simulink model "Base_Case_v1"  (R2021a)
settings: Solver=FixedStepDiscrete  StartTime=0.0  StopTime=24  FixedStep=Ts_Power  RelTol=1e-3
InitFcn:
  | %Simulation parameters
  | Ts_Power = 50e-6;
  | Ts_Control = 50e-6;
  | Ts_sec = 0.05;
  | 
  | %MV Grid parameters
  | U1n = 20e3;
  | f = 50;
  | omega = 2*pi*50;
  | 
  | 
  | %LCL filter parameters
  | L_t = 100e-6;
  | C = 173e-6;
  | L_s = 100e-6;
  | R_d = 0.086;
  | R_t = omega*L_t/100;
  | R_s = omega*L_s/100;
  | 
  | %Capacitance of the DC bus
  | Cdc = 5.88e-3;
  | Rdc = 0.00001;
  | 
  | %Coupling transformers parameters
  | U2n = 400;
  | Sn1 = 3e6;
  | 
  | %Primary Subestation parameters
  | Un = 110e3;
  | Sn = 30e6;
  | 
  | %Feeder parameters
  | Le_line_1 = 12; %length km
  | R_line_1 = (0.337)*Le_line_1; %Resistance ohms
  | X_line_1 = (0.358)*Le_line_1; %Reactance ohms
  | L_line_1 = X_line_1/omega;%Inductance H
  | 
  | Le_line_2 = 10; %length km
  | R_line_2 = (0.337)*Le_line_2; %Resistance ohms
  | X_line_2 = (0.358)*Le_line_2; %Reactance ohms
  | L_line_2 = X_line_2/omega; %Inductance H
  | 
  | %PLL parameters
  | K_p_pll = 1.8;
  | K_i_pll = 1.8/0.00251;
  | 
  | %Current control loop gains
  | tau_c = 3e-3;
  | L = L_t + L_s;
  | R =R_t + R_s;
  | Kp = L/tau_c;
  | Ki = R/tau_c;
  | 
  | %DC bus voltage control loop gains
  | tau_dc = 3*tau_c;
  | 
  | %Q-V primary control loop
  | RQ = 0.15; %Q-V regulation constant
  | 
  | %24-hours household profile pu
  | t_profile = [0:1:24].';
  | p_profile_h = [0.26 0.2 0.19 0.19 0.19 0.25 0.4 0.6 0.64 0.64 0.67 0.6 0.73 0.63 0.57 0.5 0.47 0.65 0.8 0.93 0.82 0.67 0.55 0.38 0.26].';
  | fdp_h = 0.87;
  | fi_h = acos(fdp_h);
  | q_profile_h = p_profile_h*tan(fi_h);
  | S_h = 3e6;
  | 
  | %24-hours industrial profile pu
  | p_profile_i = [0.33 0.32 0.29 0.32 0.37 0.45 0.67 0.88 1 0.99 1 0.79 0.83 0.83 0.83 0.8 0.55 0.65 0.5 0.46 0.41 0.4 0.36 0.36 0.33].';
  | fdp_i = 0.98;
  | fi_i = acos(fdp_h);
  | q_profile_i = p_profile_i*tan(fi_i);
  | S_i = 3e6;
  | 
  | %24-hours PV profile pu
  | p_profile_pv = [0 0 0 0 0 0 0 0 0 0.03 0.12 0.14 0.15 0.12 0.11 0.10 0.09 0.07 0.04 0 0 0 0 0 0].'*1/0.15;
  | S_pv = 6e6;
  | 
  | %24-hours WT profile pu
  | p_profile_wt = [0.9 0.9 1.1 1 0.9 1.1 1.25 1 0.9 0.8 0.9 0.9 1 0.8 1.5 1.3 1.2 1.2 1 0.7 1.2 0.9 1.3 1.4 0.9].'*1/1.5;
  | S_wt= 8e6;
undefined symbols (not defined in the file): DiscIntNeverNeededParam
libraries: spsThreePhaseSeriesRLCBranchLib x10, spsThreePhaseVIMeasurementLib x9, spsRMSLib x8, simulink x6, spsThreePhaseDynamicLoadLib x4, spsThreePhaseBreakerLib x2, spsThreePhaseTransformerTwoWindingsLib x2, spsThreePhaseSourceLib x1, spsPower3phInstantaneousLib x1, spspowerguiLib x1
settings Model: Creator=Manuel  LastModifiedBy=Manuel_Barragan

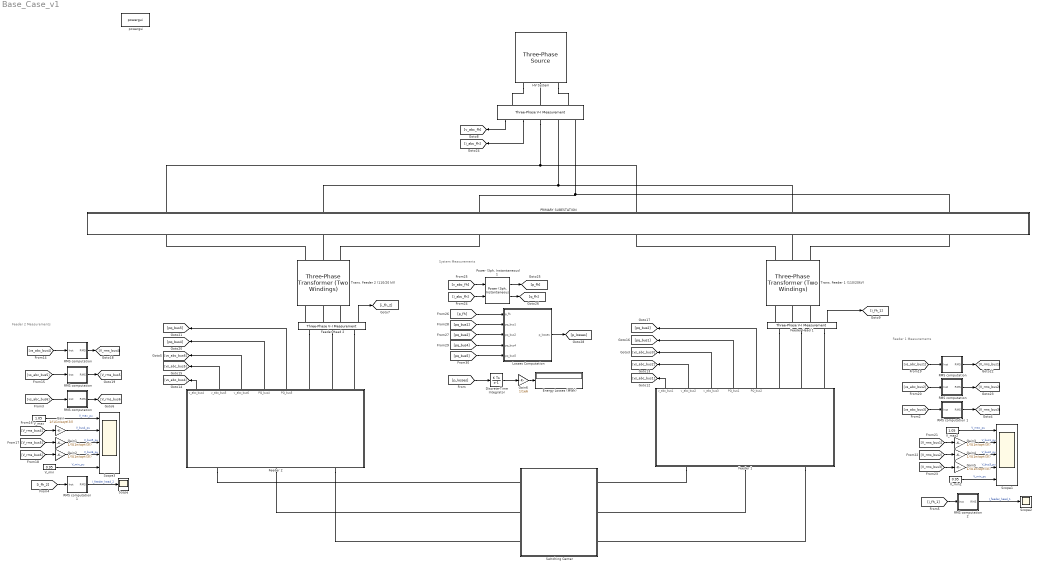
== system Base_Case_v1 ==
  note: Feeder 2 Measurements
  note: Feeder 1 Measurements
  note: System Measurements
  " " : spsThreePhaseVIMeasurementLib/Three-Phase V-I Measurement  VoltageMeasurement=phase-to-ground  SetLabelV=off  LabelV=Vabc  Vpu=off  VpuLL=off  CurrentMeasurement=yes  SetLabelI=off  LabelI=Iabc  Ipu=off  Pbase=100e6  Vbase=500e3  OutputType=Complex  PhasorSimulation=off  PSBequivalent=0
  Discrete-Time Integrator : DiscreteIntegrator  SampleTime=Ts_Control  ICPrevOutput=DiscIntNeverNeededParam  ICPrevScaledInput=DiscIntNeverNeededParam
  Energy Losses (MWh) : Display
  Feeder 1 : Subsystem
  Feeder 2 : Subsystem
  Feeder Head 1 : spsThreePhaseVIMeasurementLib/Three-Phase V-I Measurement  VoltageMeasurement=no  SetLabelV=off  LabelV=Vabc  Vpu=off  VpuLL=off  CurrentMeasurement=yes  SetLabelI=off  LabelI=Iabc  Ipu=off  Pbase=100e6  Vbase=500e3  OutputType=Complex  PhasorSimulation=off  PSBequivalent=0
  Feeder Head 2 : spsThreePhaseVIMeasurementLib/Three-Phase V-I Measurement  VoltageMeasurement=no  SetLabelV=off  LabelV=Vabc  Vpu=off  VpuLL=off  CurrentMeasurement=yes  SetLabelI=off  LabelI=Iabc  Ipu=off  Pbase=100e6  Vbase=500e3  OutputType=Complex  PhasorSimulation=off  PSBequivalent=0
  Gain{,1..5} (6 alike) : Gain  Gain=1/(U1n/sqrt(3))
  Gain6 : Gain  Gain=1/1e6
  HV System : spsThreePhaseSourceLib/Three-Phase Source  InternalConnection=Yg  VoltagePhases=off  Voltage=Un  PhaseAngle=0  Voltage_phases=[25e3 25e3 25e3]/sqrt(3)  PhaseAngles_phases=[0 -120 +120]  Frequency=f  NonIdealSource=off  SpecifyImpedance=on  Resistance=0.8929  Inductance=16.58e-3  ShortCircuitLevel=100e6  BaseVoltage=V  XRratio=7  BusType=swing  Pref=10e3  Qref=0  Prefabc=[10e3, 10e3, 10e3]  Qrefabc=[0, 0, 0]  Qmin=-inf  Qmax=inf
  Losses Computation : MATLAB Function  TreatAsAtomicUnit=on
  PRIMARY SUBESTATION : Subsystem
  "Power (3ph, Instantaneous)1" : spsPower3phInstantaneousLib/Power (3ph, Instantaneous)
  RMS computation : Subsystem
  "RMS computation " : Subsystem
  "RMS computation  " : Subsystem
  "RMS computation   " : Subsystem
  "RMS computation    " : Subsystem
  RMS computation  1 : Subsystem
  RMS computation  2 : Subsystem
  RMS computation 1 : Subsystem
  Scope : Scope
  Scope1 : Scope  NumInputPorts=5
  Scope2 : Scope
  Scope3 : Scope  NumInputPorts=5
  Switching Center : Subsystem
  Trans. Feeder 1 (110/20kV) : spsThreePhaseTransformerTwoWindingsLib/Three-Phase Transformer (Two Windings)  Winding1Connection=Yg  Winding2Connection=Yg  CoreType=Three single-phase transformers  SetSaturation=off  Hysteresis=off  DataFile='hysteresis'  SetInitialFlux=off  Measurements=None  UNITS=pu  NominalPower=[ Sn , f ]  Winding1=[ Un , 0.002 , 0.08 ]  Winding2=[ U1n , 0.002 , 0.08 ]  Rm=500  Lm=500  L0=0.5  Saturation=[ 0,0 ; 0.0024,1.2 ; 1.0,1.52 ]  InitialFluxes=[ 0.8 , -0.8 , 0.7 ]  BreakLoop=off  DiscreteSolver=Trapezoidal iterative  DataType=off  TransfoNumber=1
  Trans. Feeder 2 (110/20 kV) : spsThreePhaseTransformerTwoWindingsLib/Three-Phase Transformer (Two Windings)  Winding1Connection=Yg  Winding2Connection=Yg  CoreType=Three single-phase transformers  SetSaturation=off  Hysteresis=off  DataFile='hysteresis'  SetInitialFlux=off  Measurements=None  UNITS=pu  NominalPower=[Sn , f ]  Winding1=[ Un , 0.002 , 0.08 ]  Winding2=[ U1n , 0.002 , 0.08 ]  Rm=500  Lm=500  L0=0.5  Saturation=[ 0,0 ; 0.0024,1.2 ; 1.0,1.52 ]  InitialFluxes=[ 0.8 , -0.8 , 0.7 ]  BreakLoop=off  DiscreteSolver=Trapezoidal iterative  DataType=off  TransfoNumber=1
  V_max : Constant  Value=1.05
  V_max2 : Constant  Value=1.05
  V_min : Constant  Value=0.95
  V_min2 : Constant  Value=0.95
  powergui : spspowerguiLib/powergui  Priority=1  SimulationMode=Discrete  SampleTime=Ts_Power  frequency=60  Iterations=50  frequencyindice=50  Pbase=100e6  ErrMax=1e-4  UnitsV=kV  UnitsW=MW  buscounter=0  FunctionMessages=off  echomessages=off  EnableUseOfTLC=off  CurrentSourceSwitches=off  DisableSnubberDevices=off  DisableRonSwitches=off  DisableVfSwitches=off  DisplayEquations=off  AutomaticDiscreteSolvers=off  SolverType=Tustin/Backward Euler (TBE)  Interpol=off  ExternalGateDelay=off  methode=off  Ts=100  x0status=blocks  SPID=on  SwTol=0  HookPort=off  NonlinearTolerance=1e-4  nMaxIteration=100  ContinueOnMaxIteration=off  RestoreLinks=warning  ResistiveCurrentMeasurement=off  Frange=[0:2:500]  Ylog=off  Xlog=on  ShowGrid=off  save=off  variable=ZData  structure=0  ZoomFFT=off  StartTime=0.0  cycles=1  DisplayStyle=1  fundamental=60  FreqAxis=off  MaxFrequency=1000  frequencyindicesteady=1  RmsSteady=1  display=off
  wires:
  Feeder 1/1(v_abc_bus1) -> [vs_abc_bus1]
  Feeder 1/2(v_abc_bus2) -> [vs_abc_bus2]
  Feeder 1/4(PQ_bus1) -> [pq_bus1]
  Feeder 1/5(PQ_bus2) -> [pq_bus2]
  Feeder 2/1(v_abc_bus4) -> [vs_abc_bus4]
  Feeder 2/2(v_abc_bus5) -> [vs_abc_bus5]
  Feeder 2/4(PQ_bus4) -> [pq_bus4]
  Feeder 2/5(PQ_bus5) -> [pq_bus5]
  [vs_abc_bus4] -> "RMS computation  "/1(Inst)
  "RMS computation  "/1(RMS) -> [V_rms_bus4]
  "RMS computation   "/1(RMS) -> [V_rms_bus5]
  [vs_abc_bus5] -> "RMS computation   "/1(Inst)
  [vs_abc_bus2] -> "RMS computation "/1(Inst)
  "RMS computation "/1(RMS) -> [V_rms_bus2]
  RMS computation/1(RMS) -> [V_rms_bus1]
  [vs_abc_bus1] -> RMS computation/1(Inst)
  [V_rms_bus4] -> Gain/1
  Gain/1 -> Scope3/2  "V_bus4_pu"
  Gain1/1 -> Scope3/3  "V_bus5_pu"
  [V_rms_bus5] -> Gain1/1
  Gain2/1 -> Scope3/4  "V_bus6_pu"
  [V_rms_bus6] -> Gain2/1
  [V_rms_bus3] -> Gain5/1
  Gain5/1 -> Scope1/4  "V_bus3_pu"
  [V_rms_bus2] -> Gain4/1
  Gain4/1 -> Scope1/3  "V_bus2_pu"
  Gain3/1 -> Scope1/2  "V_bus1_pu"
  [V_rms_bus1] -> Gain3/1
  [i_abc_fh] -> "Power (3ph, Instantaneous)1"/2
  [v_abc_fh] -> "Power (3ph, Instantaneous)1"/1
  "Power (3ph, Instantaneous)1"/1 -> [p_fh]
  "Power (3ph, Instantaneous)1"/2 -> [q_fh]
  " "/1 -> [v_abc_fh]
  " "/2 -> [i_abc_fh]
  [p_fh] -> Losses Computation/1(p_fh)
  Losses Computation/1(p_losses) -> [p_losses]
  [pq_bus1] -> Losses Computation/2(pq_bus1)
  [pq_bus2] -> Losses Computation/3(pq_bus2)
  [p_losses] -> Discrete-Time Integrator/1
  Discrete-Time Integrator/1 -> Gain6/1
  Gain6/1 -> Energy Losses (MWh)/1
  Feeder 1/3(v_abc_bus3) -> [vs_abc_bus3]
  RMS computation 1/1(RMS) -> [V_rms_bus3]
  [vs_abc_bus3] -> RMS computation 1/1(Inst)
  Feeder 2/3(v_abc_bus6) -> [vs_abc_bus6]
  [pq_bus4] -> Losses Computation/4(pq_bus4)
  [pq_bus5] -> Losses Computation/5(pq_bus5)
  [vs_abc_bus6] -> "RMS computation    "/1(Inst)
  "RMS computation    "/1(RMS) -> [V_rms_bus6]
  V_max/1 -> Scope3/1  "V_max_pu"
  V_min/1 -> Scope3/5  "V_min_pu"
  V_max2/1 -> Scope1/1  "V_max_pu"
  V_min2/1 -> Scope1/5  "V_min_pu"
  Feeder Head 2/1 -> [i_fh_2]
  Feeder Head 1/1 -> [i_fh_1]
  [i_fh_2] -> RMS computation  1/1(Inst)
  RMS computation  1/1(RMS) -> Scope/1  "I_feeder_head_2"
  RMS computation  2/1(RMS) -> Scope2/1  "I_feeder_head_1"
  [i_fh_1] -> RMS computation  2/1(Inst)
  connections:
  Feeder 1/LConn1 -- Switching Center/LConn1
  Feeder 1/LConn2 -- Switching Center/LConn2
  Feeder 1/LConn3 -- Switching Center/LConn3
  Trans. Feeder 2 (110/20 kV)/LConn1 -- PRIMARY SUBESTATION/RConn1
  Trans. Feeder 2 (110/20 kV)/LConn2 -- PRIMARY SUBESTATION/RConn2
  Trans. Feeder 2 (110/20 kV)/LConn3 -- PRIMARY SUBESTATION/RConn3
  Trans. Feeder 1 (110/20kV)/LConn1 -- PRIMARY SUBESTATION/RConn4
  Trans. Feeder 1 (110/20kV)/LConn2 -- PRIMARY SUBESTATION/RConn5
  Trans. Feeder 1 (110/20kV)/LConn3 -- PRIMARY SUBESTATION/RConn6
  Feeder 2/LConn1 -- Switching Center/RConn1
  Feeder 2/LConn2 -- Switching Center/RConn2
  Feeder 2/LConn3 -- Switching Center/RConn3
  " "/LConn2 -- HV System/RConn2
  HV System/RConn1 -- " "/LConn1
  HV System/RConn3 -- " "/LConn3
  Feeder Head 2/RConn2 -- Trans. Feeder 2 (110/20 kV)/RConn2
  Feeder Head 2/RConn1 -- Trans. Feeder 2 (110/20 kV)/RConn3
  Feeder Head 2/LConn1 -- Feeder 2/RConn3
  Feeder Head 2/LConn2 -- Feeder 2/RConn2
  Feeder Head 2/LConn3 -- Feeder 2/RConn1
  Feeder Head 2/RConn3 -- Trans. Feeder 2 (110/20 kV)/RConn1
  Feeder Head 1/RConn2 -- Trans. Feeder 1 (110/20kV)/RConn2
  Feeder Head 1/RConn1 -- Trans. Feeder 1 (110/20kV)/RConn3
  Feeder Head 1/RConn3 -- Trans. Feeder 1 (110/20kV)/RConn1
  Feeder Head 1/LConn3 -- Feeder 1/RConn1
  Feeder Head 1/LConn2 -- Feeder 1/RConn2
  Feeder Head 1/LConn1 -- Feeder 1/RConn3
  " "/RConn1 -- PRIMARY SUBESTATION/LConn4 -- PRIMARY SUBESTATION/LConn1
  PRIMARY SUBESTATION/LConn2 -- PRIMARY SUBESTATION/LConn5 -- " "/RConn2
  PRIMARY SUBESTATION/LConn3 -- PRIMARY SUBESTATION/LConn6 -- " "/RConn3

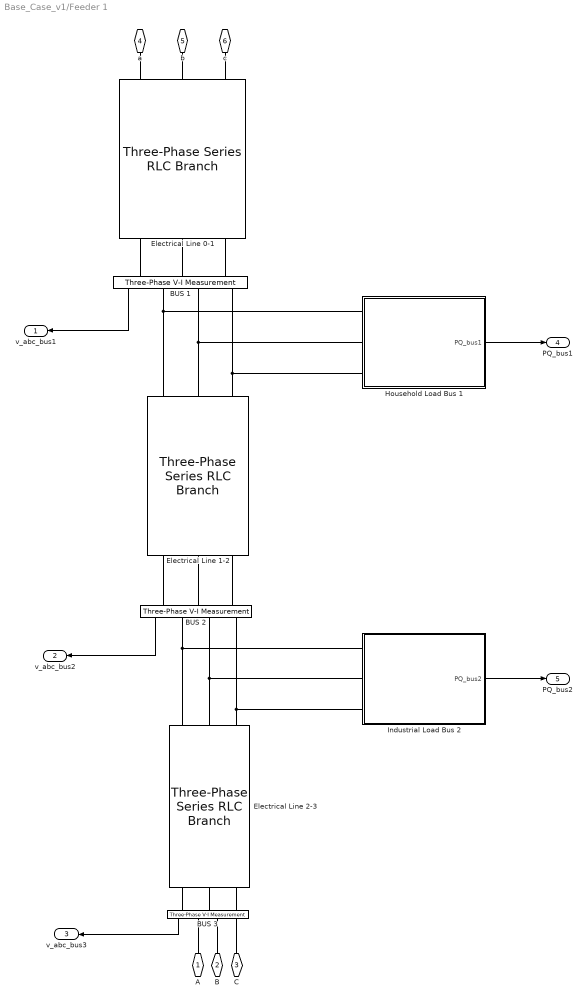
== system Base_Case_v1/Feeder 1 ==
  BUS 1 : spsThreePhaseVIMeasurementLib/Three-Phase V-I Measurement  VoltageMeasurement=phase-to-ground  SetLabelV=off  LabelV=Vabc  Vpu=off  VpuLL=off  CurrentMeasurement=no  SetLabelI=off  LabelI=Iabc  Ipu=off  Pbase=100e6  Vbase=500e3  OutputType=Complex  PhasorSimulation=off  PSBequivalent=0
  BUS 2 : spsThreePhaseVIMeasurementLib/Three-Phase V-I Measurement  VoltageMeasurement=phase-to-ground  SetLabelV=off  LabelV=Vabc  Vpu=off  VpuLL=off  CurrentMeasurement=no  SetLabelI=off  LabelI=Iabc  Ipu=off  Pbase=100e6  Vbase=500e3  OutputType=Complex  PhasorSimulation=off  PSBequivalent=0
  BUS 3 : spsThreePhaseVIMeasurementLib/Three-Phase V-I Measurement  VoltageMeasurement=phase-to-ground  SetLabelV=off  LabelV=Vabc  Vpu=off  VpuLL=off  CurrentMeasurement=no  SetLabelI=off  LabelI=Iabc  Ipu=off  Pbase=100e6  Vbase=500e3  OutputType=Complex  PhasorSimulation=off  PSBequivalent=0
  Electrical Line 0-1 : spsThreePhaseSeriesRLCBranchLib/Three-Phase Series RLC Branch  LConnTagsString=A|B|C  RConnTagsString=A|B|C  BranchType=RL  Resistance=R_line_1*0.35  Inductance=L_line_1*0.35  Capacitance=1e-6  Measurements=None
  Electrical Line 1-2 : spsThreePhaseSeriesRLCBranchLib/Three-Phase Series RLC Branch  LConnTagsString=A|B|C  RConnTagsString=A|B|C  BranchType=RL  Resistance=R_line_1/2  Inductance=L_line_1/2  Capacitance=1e-6  Measurements=None
  Electrical Line 2-3 : spsThreePhaseSeriesRLCBranchLib/Three-Phase Series RLC Branch  LConnTagsString=A|B|C  RConnTagsString=A|B|C  BranchType=RL  Resistance=R_line_1*0.15  Inductance=L_line_1*0.15  Capacitance=1e-6  Measurements=None
  Household Load Bus 1 : Subsystem
  Industrial Load Bus 2 : Subsystem
  A : PMIOPort  Side=Left
  B : PMIOPort  Port=2  Side=Left
  C : PMIOPort  Port=3  Side=Left
  a : PMIOPort  Port=4  Side=Right
  b : PMIOPort  Port=5  Side=Right
  c : PMIOPort  Port=6  Side=Right
  v_abc_bus1 : Outport
  v_abc_bus2 : Outport  Port=2
  v_abc_bus3 : Outport  Port=3
  PQ_bus1 : Outport  Port=4
  PQ_bus2 : Outport  Port=5
  wires:
  BUS 1/1 -> v_abc_bus1/1
  BUS 2/1 -> v_abc_bus2/1
  Household Load Bus 1/1(PQ_bus1) -> PQ_bus1/1
  Industrial Load Bus 2/1(PQ_bus2) -> PQ_bus2/1
  BUS 3/1 -> v_abc_bus3/1
  connections:
  b/RConn1 -- Electrical Line 0-1/RConn2
  BUS 1/LConn3 -- Electrical Line 0-1/LConn3
  a/RConn1 -- Electrical Line 0-1/RConn1
  c/RConn1 -- Electrical Line 0-1/RConn3
  BUS 1/LConn2 -- Electrical Line 0-1/LConn2
  BUS 1/LConn1 -- Electrical Line 0-1/LConn1
  BUS 2/LConn1 -- Electrical Line 1-2/LConn1
  BUS 2/LConn2 -- Electrical Line 1-2/LConn2
  BUS 2/LConn3 -- Electrical Line 1-2/LConn3
  Electrical Line 1-2/RConn1 -- Household Load Bus 1/LConn1 -- BUS 1/RConn1
  Electrical Line 1-2/RConn2 -- Household Load Bus 1/LConn2 -- BUS 1/RConn2
  Electrical Line 1-2/RConn3 -- Household Load Bus 1/LConn3 -- BUS 1/RConn3
  Electrical Line 2-3/RConn2 -- Industrial Load Bus 2/LConn2 -- BUS 2/RConn2
  Electrical Line 2-3/RConn1 -- Industrial Load Bus 2/LConn1 -- BUS 2/RConn1
  Electrical Line 2-3/RConn3 -- BUS 2/RConn3 -- Industrial Load Bus 2/LConn3
  BUS 3/LConn2 -- Electrical Line 2-3/LConn2
  BUS 3/LConn1 -- Electrical Line 2-3/LConn1
  BUS 3/LConn3 -- Electrical Line 2-3/LConn3
  C/RConn1 -- BUS 3/RConn3
  B/RConn1 -- BUS 3/RConn2
  A/RConn1 -- BUS 3/RConn1

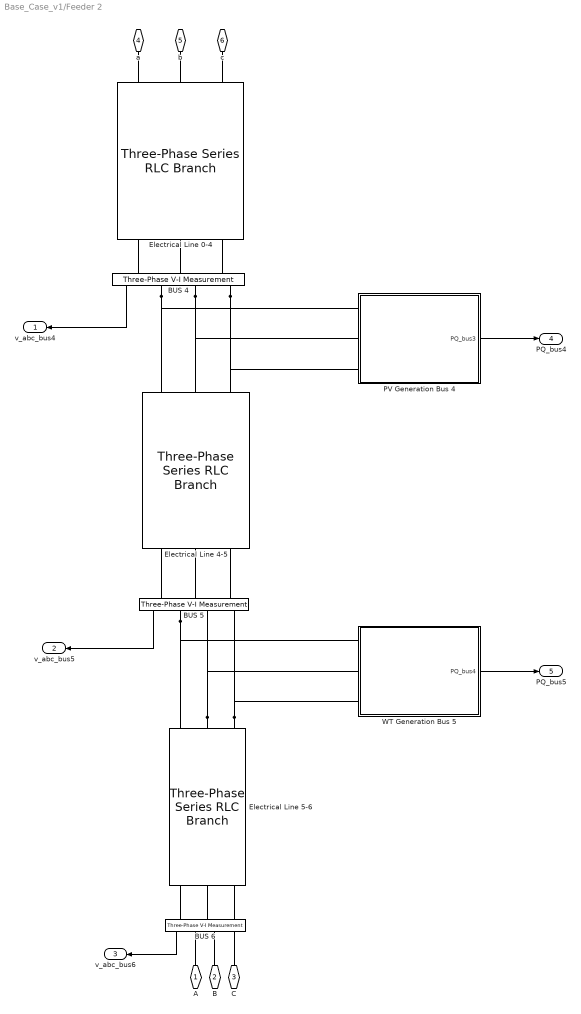
== system Base_Case_v1/Feeder 2 ==
  BUS 4 : spsThreePhaseVIMeasurementLib/Three-Phase V-I Measurement  VoltageMeasurement=phase-to-ground  SetLabelV=off  LabelV=Vabc  Vpu=off  VpuLL=off  CurrentMeasurement=no  SetLabelI=off  LabelI=Iabc  Ipu=off  Pbase=100e6  Vbase=500e3  OutputType=Complex  PhasorSimulation=off  PSBequivalent=0
  BUS 5 : spsThreePhaseVIMeasurementLib/Three-Phase V-I Measurement  VoltageMeasurement=phase-to-ground  SetLabelV=off  LabelV=Vabc  Vpu=off  VpuLL=off  CurrentMeasurement=no  SetLabelI=off  LabelI=Iabc  Ipu=off  Pbase=100e6  Vbase=500e3  OutputType=Complex  PhasorSimulation=off  PSBequivalent=0
  BUS 6 : spsThreePhaseVIMeasurementLib/Three-Phase V-I Measurement  VoltageMeasurement=phase-to-ground  SetLabelV=off  LabelV=Vabc  Vpu=off  VpuLL=off  CurrentMeasurement=no  SetLabelI=off  LabelI=Iabc  Ipu=off  Pbase=100e6  Vbase=500e3  OutputType=Complex  PhasorSimulation=off  PSBequivalent=0
  Electrical Line 0-4 : spsThreePhaseSeriesRLCBranchLib/Three-Phase Series RLC Branch  LConnTagsString=A|B|C  RConnTagsString=A|B|C  BranchType=RL  Resistance=R_line_2*0.3  Inductance=L_line_2*0.3  Capacitance=1e-6  Measurements=None
  Electrical Line 4-5 : spsThreePhaseSeriesRLCBranchLib/Three-Phase Series RLC Branch  LConnTagsString=A|B|C  RConnTagsString=A|B|C  BranchType=RL  Resistance=R_line_2*0.5  Inductance=L_line_2*0.5  Capacitance=1e-6  Measurements=None
  Electrical Line 5-6 : spsThreePhaseSeriesRLCBranchLib/Three-Phase Series RLC Branch  LConnTagsString=A|B|C  RConnTagsString=A|B|C  BranchType=RL  Resistance=R_line_2*0.2  Inductance=L_line_2*0.2  Capacitance=1e-6  Measurements=None
  PV Generation Bus 4 : Subsystem
  WT Generation Bus 5 : Subsystem
  A : PMIOPort  Side=Left
  B : PMIOPort  Port=2  Side=Left
  C : PMIOPort  Port=3  Side=Left
  a : PMIOPort  Port=4  Side=Right
  b : PMIOPort  Port=5  Side=Right
  c : PMIOPort  Port=6  Side=Right
  v_abc_bus4 : Outport
  v_abc_bus5 : Outport  Port=2
  v_abc_bus6 : Outport  Port=3
  PQ_bus4 : Outport  Port=4
  PQ_bus5 : Outport  Port=5
  wires:
  WT Generation Bus 5/1(PQ_bus4) -> PQ_bus5/1
  PV Generation Bus 4/1(PQ_bus3) -> PQ_bus4/1
  BUS 5/1 -> v_abc_bus5/1
  BUS 4/1 -> v_abc_bus4/1
  BUS 6/1 -> v_abc_bus6/1
  connections:
  BUS 5/LConn3 -- Electrical Line 4-5/LConn3
  BUS 5/LConn2 -- Electrical Line 4-5/LConn2
  BUS 5/LConn1 -- Electrical Line 4-5/LConn1
  BUS 4/RConn3 -- Electrical Line 4-5/RConn3 -- PV Generation Bus 4/LConn3
  BUS 4/RConn2 -- Electrical Line 4-5/RConn2 -- PV Generation Bus 4/LConn2
  BUS 4/RConn1 -- Electrical Line 4-5/RConn1 -- PV Generation Bus 4/LConn1
  BUS 4/LConn1 -- Electrical Line 0-4/LConn1
  BUS 4/LConn2 -- Electrical Line 0-4/LConn2
  c/RConn1 -- Electrical Line 0-4/RConn3
  a/RConn1 -- Electrical Line 0-4/RConn1
  BUS 4/LConn3 -- Electrical Line 0-4/LConn3
  b/RConn1 -- Electrical Line 0-4/RConn2
  BUS 5/RConn1 -- WT Generation Bus 5/LConn1 -- Electrical Line 5-6/RConn1
  Electrical Line 5-6/RConn3 -- BUS 5/RConn3 -- WT Generation Bus 5/LConn3
  Electrical Line 5-6/RConn2 -- BUS 5/RConn2 -- WT Generation Bus 5/LConn2
  BUS 6/LConn2 -- Electrical Line 5-6/LConn2
  BUS 6/LConn3 -- Electrical Line 5-6/LConn3
  BUS 6/LConn1 -- Electrical Line 5-6/LConn1
  BUS 6/RConn3 -- C/RConn1
  B/RConn1 -- BUS 6/RConn2
  A/RConn1 -- BUS 6/RConn1

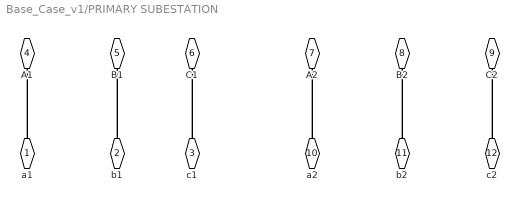
== system Base_Case_v1/PRIMARY SUBESTATION ==
  a1 : PMIOPort  Side=Right
  b1 : PMIOPort  Port=2  Side=Right
  c1 : PMIOPort  Port=3  Side=Right
  A1 : PMIOPort  Port=4  Side=Left
  B1 : PMIOPort  Port=5  Side=Left
  C1 : PMIOPort  Port=6  Side=Left
  A2 : PMIOPort  Port=7  Side=Left
  B2 : PMIOPort  Port=8  Side=Left
  C2 : PMIOPort  Port=9  Side=Left
  a2 : PMIOPort  Port=10  Side=Right
  b2 : PMIOPort  Port=11  Side=Right
  c2 : PMIOPort  Port=12  Side=Right
  connections:
  a1/RConn1 -- A1/RConn1
  b1/RConn1 -- B1/RConn1
  c1/RConn1 -- C1/RConn1
  a2/RConn1 -- A2/RConn1
  b2/RConn1 -- B2/RConn1
  c2/RConn1 -- C2/RConn1

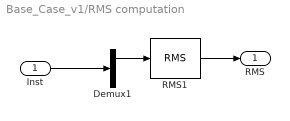
== system Base_Case_v1/RMS computation ==
  Inst : Inport
  Demux1 : Demux  Outputs=3
  RMS1 : spsRMSLib/RMS  TrueRMS=on  Freq=f  RMSInit=U2n/sqrt(3)  Ts=Ts_Control
  RMS : Outport
  wires:
  RMS1/1 -> RMS/1
  Inst/1 -> Demux1/1
  Demux1/1 -> RMS1/1

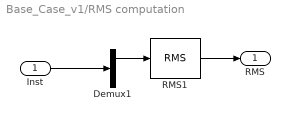
== system Base_Case_v1/RMS computation  ==
  Inst : Inport
  Demux1 : Demux  Outputs=3
  RMS1 : spsRMSLib/RMS  TrueRMS=on  Freq=f  RMSInit=U2n/sqrt(3)  Ts=Ts_Control
  RMS : Outport
  wires:
  RMS1/1 -> RMS/1
  Inst/1 -> Demux1/1
  Demux1/1 -> RMS1/1

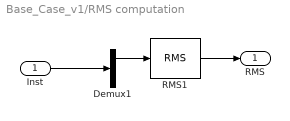
== system Base_Case_v1/RMS computation   ==
  Inst : Inport
  Demux1 : Demux  Outputs=3
  RMS1 : spsRMSLib/RMS  TrueRMS=on  Freq=f  RMSInit=U2n/sqrt(3)  Ts=Ts_Control
  RMS : Outport
  wires:
  RMS1/1 -> RMS/1
  Inst/1 -> Demux1/1
  Demux1/1 -> RMS1/1

== system Base_Case_v1/RMS computation    ==
  Inst : Inport
  Demux1 : Demux  Outputs=3
  RMS1 : spsRMSLib/RMS  TrueRMS=on  Freq=f  RMSInit=U2n/sqrt(3)  Ts=Ts_Control
  RMS : Outport
  wires:
  RMS1/1 -> RMS/1
  Inst/1 -> Demux1/1
  Demux1/1 -> RMS1/1

== system Base_Case_v1/RMS computation     ==
  Inst : Inport
  Demux1 : Demux  Outputs=3
  RMS1 : spsRMSLib/RMS  TrueRMS=on  Freq=f  RMSInit=U2n/sqrt(3)  Ts=Ts_Control
  RMS : Outport
  wires:
  Demux1/1 -> RMS1/1
  Inst/1 -> Demux1/1
  RMS1/1 -> RMS/1

== system Base_Case_v1/RMS computation  1 ==
  Inst : Inport
  Demux1 : Demux  Outputs=3
  RMS1 : spsRMSLib/RMS  TrueRMS=on  Freq=f  RMSInit=U2n/sqrt(3)  Ts=Ts_Control
  RMS : Outport
  wires:
  Demux1/1 -> RMS1/1
  Inst/1 -> Demux1/1
  RMS1/1 -> RMS/1

== system Base_Case_v1/RMS computation  2 ==
  Inst : Inport
  Demux1 : Demux  Outputs=3
  RMS1 : spsRMSLib/RMS  TrueRMS=on  Freq=f  RMSInit=U2n/sqrt(3)  Ts=Ts_Control
  RMS : Outport
  wires:
  Demux1/1 -> RMS1/1
  Inst/1 -> Demux1/1
  RMS1/1 -> RMS/1

== system Base_Case_v1/RMS computation 1 ==
  Inst : Inport
  Demux1 : Demux  Outputs=3
  RMS1 : spsRMSLib/RMS  TrueRMS=on  Freq=f  RMSInit=U2n/sqrt(3)  Ts=Ts_Control
  RMS : Outport
  wires:
  RMS1/1 -> RMS/1
  Inst/1 -> Demux1/1
  Demux1/1 -> RMS1/1

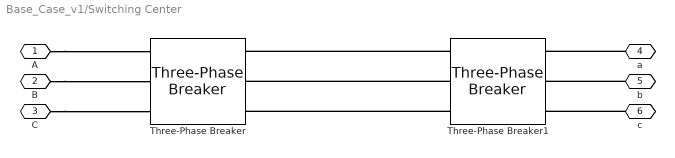
== system Base_Case_v1/Switching Center ==
  Three-Phase Breaker : spsThreePhaseBreakerLib/Three-Phase Breaker  InitialState=open  SwitchA=on  SwitchB=on  SwitchC=on  SwitchTimes="[30  31]"  External=off  BreakerResistance=0.01  SnubberResistance=1e6  SnubberCapacitance=inf  Measurements=None
  Three-Phase Breaker1 : spsThreePhaseBreakerLib/Three-Phase Breaker  InitialState=open  SwitchA=on  SwitchB=on  SwitchC=on  SwitchTimes="[30  31]"  External=off  BreakerResistance=0.01  SnubberResistance=1e6  SnubberCapacitance=inf  Measurements=None
  A : PMIOPort  Side=Right
  B : PMIOPort  Port=2  Side=Right
  C : PMIOPort  Port=3  Side=Right
  a : PMIOPort  Port=4  Side=Left
  b : PMIOPort  Port=5  Side=Left
  c : PMIOPort  Port=6  Side=Left
  connections:
  A/RConn1 -- Three-Phase Breaker/LConn1
  B/RConn1 -- Three-Phase Breaker/LConn2
  C/RConn1 -- Three-Phase Breaker/LConn3
  Three-Phase Breaker1/LConn2 -- Three-Phase Breaker/RConn2
  Three-Phase Breaker1/LConn3 -- Three-Phase Breaker/RConn3
  Three-Phase Breaker1/LConn1 -- Three-Phase Breaker/RConn1
  a/RConn1 -- Three-Phase Breaker1/RConn1
  b/RConn1 -- Three-Phase Breaker1/RConn2
  c/RConn1 -- Three-Phase Breaker1/RConn3

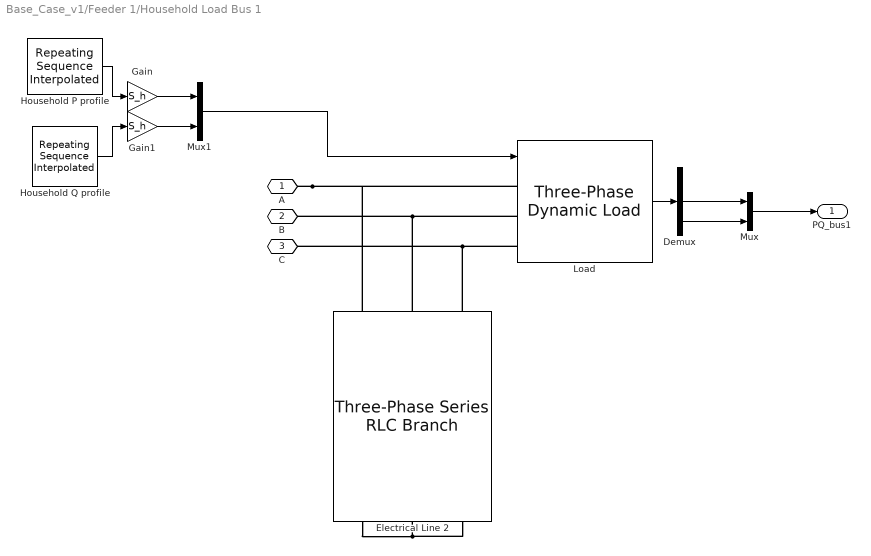
== system Base_Case_v1/Feeder 1/Household Load Bus 1 ==
  Demux : Demux  Outputs=3
  Electrical Line 2 : spsThreePhaseSeriesRLCBranchLib/Three-Phase Series RLC Branch  LConnTagsString=A|B|C  RConnTagsString=A|B|C  BranchType=R  Resistance=1e6  Inductance=L_line_2/2  Capacitance=1e-6  Measurements=None
  Gain : Gain  Gain=S_h
  Gain1 : Gain  Gain=S_h
  Household P profile : simulink/Sources/Repeating Sequence Interpolated  OutValues=p_profile_h  TimeValues=t_profile  LookUpMeth=Interpolation-Use End Values  tsamp=Ts_Control  OutMin=[]  OutMax=[]  OutDataTypeStr=double  OutputDataTypeScalingMode=double  OutDataType=fixdt(0,8)  OutScaling=2^-10
  Household Q profile : simulink/Sources/Repeating Sequence Interpolated  OutValues=q_profile_h  TimeValues=t_profile  LookUpMeth=Interpolation-Use End Values  tsamp=Ts_Control  OutMin=[]  OutMax=[]  OutDataTypeStr=double  OutputDataTypeScalingMode=double  OutDataType=fixdt(0,8)  OutScaling=2^-10
  Load : spsThreePhaseDynamicLoadLib/Three-Phase Dynamic Load  NominalVoltage=[U1n f ]  ActiveReactivePowers=[0 0]  PositiveSequence=[1 0]  ExternalControl=on  NpNq=[1.3 2]  TimeConstants="[0  0  0  0]"  MinimumVoltage=0.7  Tfilter=1e-4  LoadFlowParameters=[4,0,0,0,0]
      settings: SourceProductBaseCode=PS
  Mux : Mux  Inputs=2
  Mux1 : Mux  Inputs=2
  A : PMIOPort  Side=Left
  B : PMIOPort  Port=2  Side=Left
  C : PMIOPort  Port=3  Side=Left
  PQ_bus1 : Outport
  wires:
  Load/1 -> Demux/1
  Demux/2 -> Mux/1
  Demux/3 -> Mux/2
  Mux/1 -> PQ_bus1/1
  Household P profile/1 -> Gain/1
  Gain/1 -> Mux1/1
  Gain1/1 -> Mux1/2
  Household Q profile/1 -> Gain1/1
  Mux1/1 -> Load/1
  connections:
  Electrical Line 2/LConn2 -- Load/LConn2 -- B/RConn1
  Electrical Line 2/LConn3 -- Load/LConn3 -- C/RConn1
  A/RConn1 -- Load/LConn1 -- Electrical Line 2/LConn1
  Electrical Line 2/RConn2 -- Electrical Line 2/RConn1 -- Electrical Line 2/RConn3

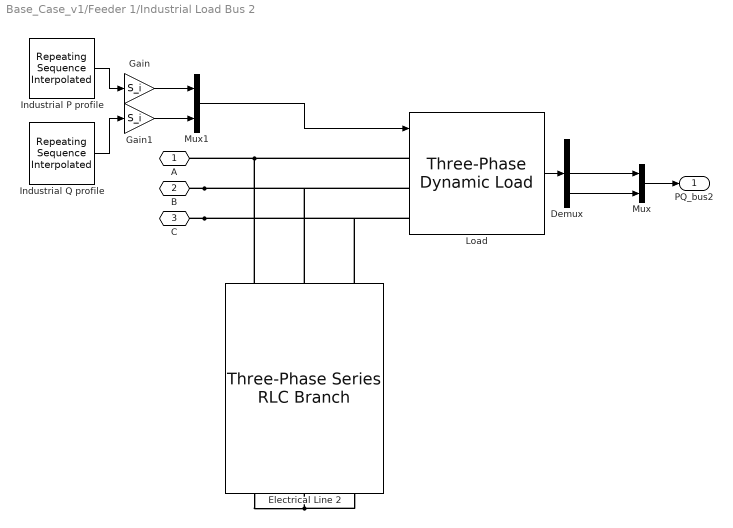
== system Base_Case_v1/Feeder 1/Industrial Load Bus 2 ==
  Demux : Demux  Outputs=3
  Electrical Line 2 : spsThreePhaseSeriesRLCBranchLib/Three-Phase Series RLC Branch  LConnTagsString=A|B|C  RConnTagsString=A|B|C  BranchType=R  Resistance=1e6  Inductance=L_line_2/2  Capacitance=1e-6  Measurements=None
  Gain : Gain  Gain=S_i
  Gain1 : Gain  Gain=S_i
  Industrial P profile : simulink/Sources/Repeating Sequence Interpolated  OutValues=p_profile_i  TimeValues=t_profile  LookUpMeth=Interpolation-Use End Values  tsamp=Ts_Control  OutMin=[]  OutMax=[]  OutDataTypeStr=double  OutputDataTypeScalingMode=double  OutDataType=fixdt(0,8)  OutScaling=2^-10
  Industrial Q profile : simulink/Sources/Repeating Sequence Interpolated  OutValues=q_profile_i  TimeValues=t_profile  LookUpMeth=Interpolation-Use End Values  tsamp=Ts_Control  OutMin=[]  OutMax=[]  OutDataTypeStr=double  OutputDataTypeScalingMode=double  OutDataType=fixdt(0,8)  OutScaling=2^-10
  Load : spsThreePhaseDynamicLoadLib/Three-Phase Dynamic Load  NominalVoltage=[U1n f ]  ActiveReactivePowers=[0 0]  PositiveSequence=[1 0]  ExternalControl=on  NpNq=[1.3 2]  TimeConstants="[0  0  0  0]"  MinimumVoltage=0.7  Tfilter=1e-4  LoadFlowParameters=[4,0,0,0,0]
      settings: SourceProductBaseCode=PS
  Mux : Mux  Inputs=2
  Mux1 : Mux  Inputs=2
  A : PMIOPort  Side=Left
  B : PMIOPort  Port=2  Side=Left
  C : PMIOPort  Port=3  Side=Left
  PQ_bus2 : Outport
  wires:
  Load/1 -> Demux/1
  Mux/1 -> PQ_bus2/1
  Demux/3 -> Mux/2
  Demux/2 -> Mux/1
  Gain/1 -> Mux1/1
  Industrial P profile/1 -> Gain/1
  Gain1/1 -> Mux1/2
  Industrial Q profile/1 -> Gain1/1
  Mux1/1 -> Load/1
  connections:
  Electrical Line 2/RConn3 -- Electrical Line 2/RConn1 -- Electrical Line 2/RConn2
  Electrical Line 2/LConn1 -- Load/LConn1 -- A/RConn1
  C/RConn1 -- Load/LConn3 -- Electrical Line 2/LConn3
  B/RConn1 -- Load/LConn2 -- Electrical Line 2/LConn2

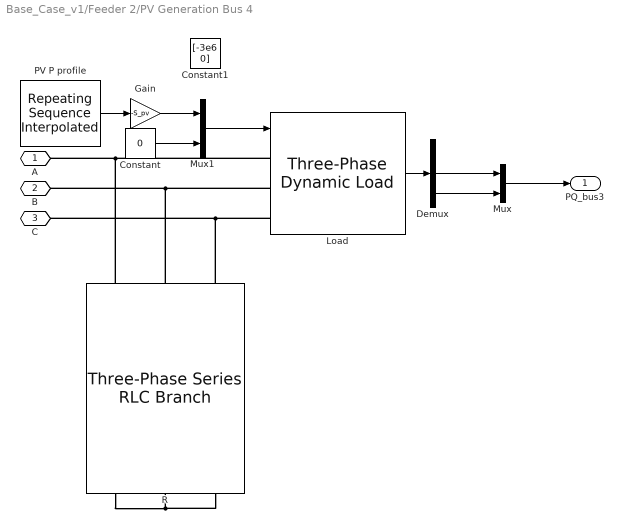
== system Base_Case_v1/Feeder 2/PV Generation Bus 4 ==
  Constant : Constant  Value=0
  Constant1 : Constant  Value=[-3e6 0]
  Demux : Demux  Outputs=3
  Gain : Gain  Gain=-S_pv
  Load : spsThreePhaseDynamicLoadLib/Three-Phase Dynamic Load  NominalVoltage=[U1n f ]  ActiveReactivePowers=[0 0]  PositiveSequence=[1 0]  ExternalControl=on  NpNq=[1.3 2]  TimeConstants="[0  0  0  0]"  MinimumVoltage=0.7  Tfilter=1e-4  LoadFlowParameters=[4,0,0,0,0]
      settings: SourceProductBaseCode=PS
  Mux : Mux  Inputs=2
  Mux1 : Mux  Inputs=2
  PV P profile : simulink/Sources/Repeating Sequence Interpolated  OutValues=p_profile_pv  TimeValues=t_profile  LookUpMeth=Interpolation-Use End Values  tsamp=Ts_Control  OutMin=[]  OutMax=[]  OutDataTypeStr=double  OutputDataTypeScalingMode=double  OutDataType=fixdt(0,8)  OutScaling=2^-10
  R : spsThreePhaseSeriesRLCBranchLib/Three-Phase Series RLC Branch  LConnTagsString=A|B|C  RConnTagsString=A|B|C  BranchType=R  Resistance=1e6  Inductance=L_line_2/2  Capacitance=1e-6  Measurements=None
  A : PMIOPort  Side=Left
  B : PMIOPort  Port=2  Side=Left
  C : PMIOPort  Port=3  Side=Left
  PQ_bus3 : Outport
  wires:
  Mux/1 -> PQ_bus3/1
  Demux/3 -> Mux/2
  Demux/2 -> Mux/1
  Load/1 -> Demux/1
  PV P profile/1 -> Gain/1
  Gain/1 -> Mux1/1
  Constant/1 -> Mux1/2
  Mux1/1 -> Load/1
  connections:
  R/RConn3 -- R/RConn1 -- R/RConn2
  Load/LConn1 -- R/LConn1 -- A/RConn1
  Load/LConn3 -- R/LConn3 -- C/RConn1
  Load/LConn2 -- R/LConn2 -- B/RConn1

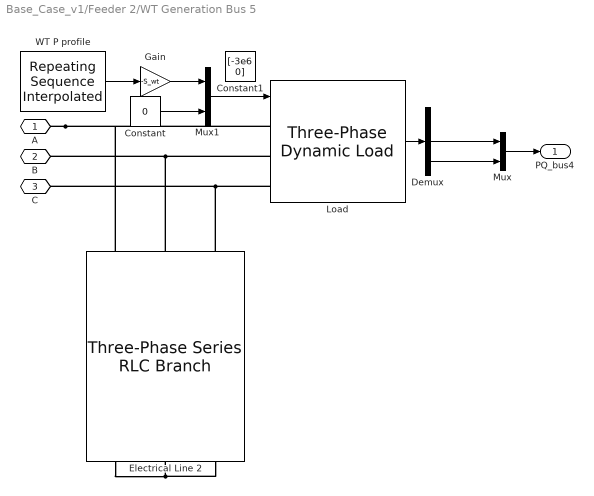
== system Base_Case_v1/Feeder 2/WT Generation Bus 5 ==
  Constant : Constant  Value=0
  Constant1 : Constant  Value=[-3e6 0]
  Demux : Demux  Outputs=3
  Electrical Line 2 : spsThreePhaseSeriesRLCBranchLib/Three-Phase Series RLC Branch  LConnTagsString=A|B|C  RConnTagsString=A|B|C  BranchType=R  Resistance=1e6  Inductance=L_line_2/2  Capacitance=1e-6  Measurements=None
  Gain : Gain  Gain=-S_wt
  Load : spsThreePhaseDynamicLoadLib/Three-Phase Dynamic Load  NominalVoltage=[U1n f ]  ActiveReactivePowers=[0 0]  PositiveSequence=[1 0]  ExternalControl=on  NpNq=[1.3 2]  TimeConstants="[0  0  0  0]"  MinimumVoltage=0.7  Tfilter=1e-4  LoadFlowParameters=[4,0,0,0,0]
      settings: SourceProductBaseCode=PS
  Mux : Mux  Inputs=2
  Mux1 : Mux  Inputs=2
  WT P profile : simulink/Sources/Repeating Sequence Interpolated  OutValues=p_profile_wt  TimeValues=t_profile  LookUpMeth=Interpolation-Use End Values  tsamp=Ts_Control  OutMin=[]  OutMax=[]  OutDataTypeStr=double  OutputDataTypeScalingMode=double  OutDataType=fixdt(0,8)  OutScaling=2^-10
  A : PMIOPort  Side=Left
  B : PMIOPort  Port=2  Side=Left
  C : PMIOPort  Port=3  Side=Left
  PQ_bus4 : Outport
  wires:
  Demux/2 -> Mux/1
  Demux/3 -> Mux/2
  Mux/1 -> PQ_bus4/1
  Load/1 -> Demux/1
  WT P profile/1 -> Gain/1
  Gain/1 -> Mux1/1
  Constant/1 -> Mux1/2
  Mux1/1 -> Load/1
  connections:
  Electrical Line 2/LConn2 -- Load/LConn2 -- B/RConn1
  Electrical Line 2/LConn3 -- Load/LConn3 -- C/RConn1
  A/RConn1 -- Load/LConn1 -- Electrical Line 2/LConn1
  Electrical Line 2/RConn2 -- Electrical Line 2/RConn1 -- Electrical Line 2/RConn3

== matlab function Base_Case_v1/Losses Computation ==
  data: p_fh input; p_losses output; pq_bus1 input; pq_bus2 input; pq_bus4 input; pq_bus5 input
function p_losses = fcn(p_fh,pq_bus1,pq_bus2,pq_bus4,pq_bus5)
p_bus1=pq_bus1(1); %Load Bus1
p_bus2=pq_bus2(1); %Load Bus2
p_bus4=-pq_bus4(1); %Gen Bus3
p_bus5=-pq_bus5(1); %Gen Bus4

p_losses = abs((p_fh + p_bus4 + p_bus5) - (p_bus1+p_bus2));
